simulink model "GS_model"  (R2018b)
settings: Solver=ode5  StartTime=0.0  StopTime=SimuStopTime  FixedStep=T_Simu  RelTol=1e-3
InitFcn:
  | Initial
undefined symbols (not defined in the file or in its folder): Aba10, Aba20, aeroCIP2006_S, aeroCIP2006_X, aeroCIP2006_Y, Agl0, Ass_kS, Ass_n1, Ass_n2, Ass_n3, Ass_n4, Ass_Noise, Ass_R, Ass_Resolution, Ass_TmOrder, AssA_Fix_Abs, AssB_Fix_Abs, AssC_Fix_Abs, AssD_Fix_Abs, AssE_Fix_Aps, AssF_Fix_Aps, C, c_max, c_min, Cd, CenterOfFigNX, CenterOfFigNY, CenterOfFigNZ, CenterOfFigP1, CenterOfFigP2, CenterOfFigPX, CenterOfFigPY, CenterOfFigPZ, Cmu, Crou, DEG2RAD, DiscIntNeverNeededParam, Eg_Dir, Eg_F, Eg_PrepareTime, Eg_r_L_L, Fw_Abf, Fw_Hmax, Fw_J, Fw_Spd0, Fw_Tmax, git_hash_BaseLine, git_hash_Project, Gnss_Noise_Pos, Gnss_Noise_Vel, Gnss_PropgationTime, GyroA_Fix_Abg, GyroA_Noise, GyroB_Fix_Abg, GyroB_Noise, GyroC_Fix_Abg, GyroC_Noise, GyroD_Fix_Abg, GyroD_Noise, h ... (+94)
libraries: simulink x308, sharedutil x46, aerolibutil x37, sharedtransform x31, vrlib x14, aerolibgravity2 x2
(part 10 of 20)

== system GS_model/Subsystem2/Subsystem/Actuator/FlyWheel/FwAModel4/FWMath&ErrModel/Subsystem1 ==
  Fb_FW_T : Inport
  TC_FW_TSet : Inport  Port=2
  FWNum : Inport  Port=3
  TC_FWErr_TOp : Inport  Port=4
  Compare To Constant : simulink/Logic and Bit Operations/Compare To Constant  relop===  const=0  OutDataTypeStr=boolean
  Compare To Constant1 : simulink/Logic and Bit Operations/Compare To Constant  relop===  const=0  OutDataTypeStr=boolean
  Demux : Demux  Outputs=[1;2]
  Demux1 : Demux  Outputs=2
  Demux2 : Demux  Outputs=2
  If : If  IfExpression=u1 == 1
  If Action Subsystem : Subsystem  TreatAsAtomicUnit=on
  If Action Subsystem1 : Subsystem  TreatAsAtomicUnit=on
  Logical Operator : Logic  Operator=OR  AllPortsSameDT=off  OutDataTypeStr=boolean
  Logical Operator1 : Logic  Operator=OR  AllPortsSameDT=off  OutDataTypeStr=boolean
  Merge : Merge
  Relational Operator1 : RelationalOperator  Operator===  OutDataTypeStr=boolean  RndMeth=Simplest
  Relational Operator3 : RelationalOperator  Operator===  OutDataTypeStr=boolean  RndMeth=Simplest
  Sum : Sum  Inputs=|++
  Triggered Subsystem1 : Subsystem  TreatAsAtomicUnit=on
      mask Display: disp('FWChoice')
  Triggered Subsystem2 : Subsystem  TreatAsAtomicUnit=on
      mask Display: disp('FWChoice')
  TM_FW_T : Outport
  wires:
  FWNum/1 -> Relational Operator3/1, Relational Operator1/1
  Compare To Constant1/1 -> Logical Operator1/1
  Relational Operator1/1 -> Logical Operator1/2
  Demux2/1 -> Compare To Constant1/1, Relational Operator1/2
  Logical Operator1/1 -> Triggered Subsystem2/Enable
  Logical Operator/1 -> Triggered Subsystem1/Enable
  Demux/1 -> Relational Operator3/2, Compare To Constant/1
  Relational Operator3/1 -> Logical Operator/2
  Compare To Constant/1 -> Logical Operator/1
  Demux1/1 -> If/1
  If Action Subsystem/1(Out1) -> Merge/1
  Triggered Subsystem1/1(Out1) -> Demux1/1
  Demux/2 -> Triggered Subsystem1/1(In1)
  If/1 -> If Action Subsystem/Action
  TC_FW_TSet/1 -> Demux/1
  Sum/1 -> If Action Subsystem1/1(In1)
  Merge/1 -> TM_FW_T/1
  TC_FWErr_TOp/1 -> Demux2/1
  Demux2/2 -> Triggered Subsystem2/1(In1)
  Triggered Subsystem2/1(Out1) -> Sum/1
  If Action Subsystem1/1(Out1) -> Merge/2
  Demux1/2 -> If Action Subsystem/1(In1)
  If/2 -> If Action Subsystem1/Action
  Fb_FW_T/1 -> Sum/2

== system GS_model/Subsystem2/Subsystem/Actuator/FlyWheel/FwAModel4/FWMath&ErrModel/Subsystem2 ==
  Fb_FW_Spd : Inport
  TC_FW_SpdSet : Inport  Port=2
  FWNum : Inport  Port=3
  TC_FWErr_SpdOp : Inport  Port=4
  Compare To Constant : simulink/Logic and Bit Operations/Compare To Constant  relop===  const=0  OutDataTypeStr=boolean
  Compare To Constant1 : simulink/Logic and Bit Operations/Compare To Constant  relop===  const=0  OutDataTypeStr=boolean
  Demux : Demux  Outputs=[1;2]
  Demux1 : Demux  Outputs=2
  Demux2 : Demux  Outputs=2
  If : If  IfExpression=u1 == 1
  If Action Subsystem : Subsystem  TreatAsAtomicUnit=on
  If Action Subsystem1 : Subsystem  TreatAsAtomicUnit=on
  Logical Operator : Logic  Operator=OR  AllPortsSameDT=off  OutDataTypeStr=boolean
  Logical Operator1 : Logic  Operator=OR  AllPortsSameDT=off  OutDataTypeStr=boolean
  Merge : Merge
  Relational Operator1 : RelationalOperator  Operator===  OutDataTypeStr=boolean  RndMeth=Simplest
  Relational Operator2 : RelationalOperator  Operator===  OutDataTypeStr=boolean  RndMeth=Simplest
  Sum : Sum  Inputs=|++
  Triggered Subsystem1 : Subsystem  TreatAsAtomicUnit=on
      mask Display: disp('FWChoice')
  Triggered Subsystem2 : Subsystem  TreatAsAtomicUnit=on
      mask Display: disp('FWChoice')
  TM_FW_Spd : Outport
  wires:
  Logical Operator1/1 -> Triggered Subsystem2/Enable
  Compare To Constant1/1 -> Logical Operator1/1
  Relational Operator2/1 -> Logical Operator1/2
  Logical Operator/1 -> Triggered Subsystem1/Enable
  Compare To Constant/1 -> Logical Operator/1
  Relational Operator1/1 -> Logical Operator/2
  If/2 -> If Action Subsystem1/Action
  If Action Subsystem/1(Out1) -> Merge/1
  Demux2/1 -> Relational Operator2/2, Compare To Constant1/1
  FWNum/1 -> Relational Operator1/1, Relational Operator2/1
  Triggered Subsystem1/1(Out1) -> Demux1/1
  Fb_FW_Spd/1 -> Sum/2
  Demux/2 -> Triggered Subsystem1/1(In1)
  If Action Subsystem1/1(Out1) -> Merge/2
  Demux1/1 -> If/1
  Demux2/2 -> Triggered Subsystem2/1(In1)
  Demux1/2 -> If Action Subsystem/1(In1)
  Sum/1 -> If Action Subsystem1/1(In1)
  Triggered Subsystem2/1(Out1) -> Sum/1
  TC_FWErr_SpdOp/1 -> Demux2/1
  If/1 -> If Action Subsystem/Action
  Merge/1 -> TM_FW_Spd/1
  Demux/1 -> Relational Operator1/2, Compare To Constant/1
  TC_FW_SpdSet/1 -> Demux/1

== system GS_model/Subsystem2/Subsystem/Actuator/FlyWheel/FwAModel4/FWMath&ErrModel/Subsystem4 ==
  FWNum : Inport
  FW_Mode : Inport  Port=2
  TC_FW_ModeSet : Inport  Port=3
  Compare To Constant : simulink/Logic and Bit Operations/Compare To Constant  relop===  const=0  OutDataTypeStr=boolean
  Demux : Demux  Outputs=[1;2]
  Demux1 : Demux  Outputs=2
  If : If  IfExpression=u1 == 1
  If Action Subsystem : Subsystem  TreatAsAtomicUnit=on
  If Action Subsystem1 : Subsystem  TreatAsAtomicUnit=on
  Logical Operator : Logic  Operator=OR  AllPortsSameDT=off  OutDataTypeStr=boolean
  Merge : Merge
  Relational Operator1 : RelationalOperator  Operator===  OutDataTypeStr=boolean  RndMeth=Simplest
  Triggered Subsystem1 : Subsystem  TreatAsAtomicUnit=on
      mask Display: disp('FWChoice')
  Fb_FW_Mode : Outport
  wires:
  Compare To Constant/1 -> Logical Operator/1
  Logical Operator/1 -> Triggered Subsystem1/Enable
  Relational Operator1/1 -> Logical Operator/2
  TC_FW_ModeSet/1 -> Demux/1
  FWNum/1 -> Relational Operator1/1
  Demux/2 -> Triggered Subsystem1/1(In1)
  Demux/1 -> Relational Operator1/2, Compare To Constant/1
  Demux1/1 -> If/1
  If/1 -> If Action Subsystem/Action
  Demux1/2 -> If Action Subsystem/1(In1)
  Triggered Subsystem1/1(Out1) -> Demux1/1
  If/2 -> If Action Subsystem1/Action
  FW_Mode/1 -> If Action Subsystem1/1(In1)
  If Action Subsystem/1(Out1) -> Merge/1
  If Action Subsystem1/1(Out1) -> Merge/2
  Merge/1 -> Fb_FW_Mode/1

== system GS_model/Subsystem2/Subsystem/Actuator/FlyWheel/FwAModel5/FWDataSourceChoice/DelayModel ==
  TC_FW_Delay : Inport
  FW_Cmd_Mode : Inport  Port=2
  FW_Cmd_Spd : Inport  Port=3
  FW_Cmd_T : Inport  Port=4
  Constant3 : Constant
  Sum8 : Sum  Inputs=|++
  delay1 : Subsystem
  delay2 : Subsystem
  delay3 : Subsystem
  Cmd_Mode : Outport
  Cmd_Spd : Outport  Port=2
  Cmd_T : Outport  Port=3
  wires:
  delay2/1(Out1) -> Cmd_T/1
  FW_Cmd_T/1 -> delay2/2(In2)
  delay1/1(Out1) -> Cmd_Spd/1
  Sum8/1 -> delay1/1(In1), delay2/1(In1), delay3/1(In1)
  FW_Cmd_Spd/1 -> delay1/2(In2)
  Constant3/1 -> Sum8/2
  TC_FW_Delay/1 -> Sum8/1
  FW_Cmd_Mode/1 -> delay3/2(In2)
  delay3/1(Out1) -> Cmd_Mode/1

== system GS_model/Subsystem2/Subsystem/Actuator/FlyWheel/FwAModel5/FWMath&ErrModel/Subsystem1 ==
  Fb_FW_T : Inport
  TC_FW_TSet : Inport  Port=2
  FWNum : Inport  Port=3
  TC_FWErr_TOp : Inport  Port=4
  Compare To Constant : simulink/Logic and Bit Operations/Compare To Constant  relop===  const=0  OutDataTypeStr=boolean
  Compare To Constant1 : simulink/Logic and Bit Operations/Compare To Constant  relop===  const=0  OutDataTypeStr=boolean
  Demux : Demux  Outputs=[1;2]
  Demux1 : Demux  Outputs=2
  Demux2 : Demux  Outputs=2
  If : If  IfExpression=u1 == 1
  If Action Subsystem : Subsystem  TreatAsAtomicUnit=on
  If Action Subsystem1 : Subsystem  TreatAsAtomicUnit=on
  Logical Operator : Logic  Operator=OR  AllPortsSameDT=off  OutDataTypeStr=boolean
  Logical Operator1 : Logic  Operator=OR  AllPortsSameDT=off  OutDataTypeStr=boolean
  Merge : Merge
  Relational Operator1 : RelationalOperator  Operator===  OutDataTypeStr=boolean  RndMeth=Simplest
  Relational Operator3 : RelationalOperator  Operator===  OutDataTypeStr=boolean  RndMeth=Simplest
  Sum : Sum  Inputs=|++
  Triggered Subsystem1 : Subsystem  TreatAsAtomicUnit=on
      mask Display: disp('FWChoice')
  Triggered Subsystem2 : Subsystem  TreatAsAtomicUnit=on
      mask Display: disp('FWChoice')
  TM_FW_T : Outport
  wires:
  Fb_FW_T/1 -> Sum/2
  If/2 -> If Action Subsystem1/Action
  Demux1/2 -> If Action Subsystem/1(In1)
  If Action Subsystem1/1(Out1) -> Merge/2
  Triggered Subsystem2/1(Out1) -> Sum/1
  Demux2/2 -> Triggered Subsystem2/1(In1)
  TC_FWErr_TOp/1 -> Demux2/1
  Merge/1 -> TM_FW_T/1
  Sum/1 -> If Action Subsystem1/1(In1)
  TC_FW_TSet/1 -> Demux/1
  If/1 -> If Action Subsystem/Action
  Demux/2 -> Triggered Subsystem1/1(In1)
  Triggered Subsystem1/1(Out1) -> Demux1/1
  If Action Subsystem/1(Out1) -> Merge/1
  Demux1/1 -> If/1
  Compare To Constant/1 -> Logical Operator/1
  Relational Operator3/1 -> Logical Operator/2
  Demux/1 -> Compare To Constant/1, Relational Operator3/2
  Logical Operator/1 -> Triggered Subsystem1/Enable
  Logical Operator1/1 -> Triggered Subsystem2/Enable
  Demux2/1 -> Relational Operator1/2, Compare To Constant1/1
  Relational Operator1/1 -> Logical Operator1/2
  Compare To Constant1/1 -> Logical Operator1/1
  FWNum/1 -> Relational Operator1/1, Relational Operator3/1

== system GS_model/Subsystem2/Subsystem/Actuator/FlyWheel/FwAModel5/FWMath&ErrModel/Subsystem2 ==
  Fb_FW_Spd : Inport
  TC_FW_SpdSet : Inport  Port=2
  FWNum : Inport  Port=3
  TC_FWErr_SpdOp : Inport  Port=4
  Compare To Constant : simulink/Logic and Bit Operations/Compare To Constant  relop===  const=0  OutDataTypeStr=boolean
  Compare To Constant1 : simulink/Logic and Bit Operations/Compare To Constant  relop===  const=0  OutDataTypeStr=boolean
  Demux : Demux  Outputs=[1;2]
  Demux1 : Demux  Outputs=2
  Demux2 : Demux  Outputs=2
  If : If  IfExpression=u1 == 1
  If Action Subsystem : Subsystem  TreatAsAtomicUnit=on
  If Action Subsystem1 : Subsystem  TreatAsAtomicUnit=on
  Logical Operator : Logic  Operator=OR  AllPortsSameDT=off  OutDataTypeStr=boolean
  Logical Operator1 : Logic  Operator=OR  AllPortsSameDT=off  OutDataTypeStr=boolean
  Merge : Merge
  Relational Operator1 : RelationalOperator  Operator===  OutDataTypeStr=boolean  RndMeth=Simplest
  Relational Operator2 : RelationalOperator  Operator===  OutDataTypeStr=boolean  RndMeth=Simplest
  Sum : Sum  Inputs=|++
  Triggered Subsystem1 : Subsystem  TreatAsAtomicUnit=on
      mask Display: disp('FWChoice')
  Triggered Subsystem2 : Subsystem  TreatAsAtomicUnit=on
      mask Display: disp('FWChoice')
  TM_FW_Spd : Outport
  wires:
  TC_FW_SpdSet/1 -> Demux/1
  Demux/1 -> Compare To Constant/1, Relational Operator1/2
  Merge/1 -> TM_FW_Spd/1
  If/1 -> If Action Subsystem/Action
  TC_FWErr_SpdOp/1 -> Demux2/1
  Triggered Subsystem2/1(Out1) -> Sum/1
  Sum/1 -> If Action Subsystem1/1(In1)
  Demux1/2 -> If Action Subsystem/1(In1)
  Demux2/2 -> Triggered Subsystem2/1(In1)
  Demux1/1 -> If/1
  If Action Subsystem1/1(Out1) -> Merge/2
  Demux/2 -> Triggered Subsystem1/1(In1)
  Fb_FW_Spd/1 -> Sum/2
  Triggered Subsystem1/1(Out1) -> Demux1/1
  FWNum/1 -> Relational Operator2/1, Relational Operator1/1
  Demux2/1 -> Compare To Constant1/1, Relational Operator2/2
  If Action Subsystem/1(Out1) -> Merge/1
  If/2 -> If Action Subsystem1/Action
  Relational Operator1/1 -> Logical Operator/2
  Compare To Constant/1 -> Logical Operator/1
  Logical Operator/1 -> Triggered Subsystem1/Enable
  Relational Operator2/1 -> Logical Operator1/2
  Compare To Constant1/1 -> Logical Operator1/1
  Logical Operator1/1 -> Triggered Subsystem2/Enable

== system GS_model/Subsystem2/Subsystem/Actuator/FlyWheel/FwAModel5/FWMath&ErrModel/Subsystem4 ==
  FWNum : Inport
  FW_Mode : Inport  Port=2
  TC_FW_ModeSet : Inport  Port=3
  Compare To Constant : simulink/Logic and Bit Operations/Compare To Constant  relop===  const=0  OutDataTypeStr=boolean
  Demux : Demux  Outputs=[1;2]
  Demux1 : Demux  Outputs=2
  If : If  IfExpression=u1 == 1
  If Action Subsystem : Subsystem  TreatAsAtomicUnit=on
  If Action Subsystem1 : Subsystem  TreatAsAtomicUnit=on
  Logical Operator : Logic  Operator=OR  AllPortsSameDT=off  OutDataTypeStr=boolean
  Merge : Merge
  Relational Operator1 : RelationalOperator  Operator===  OutDataTypeStr=boolean  RndMeth=Simplest
  Triggered Subsystem1 : Subsystem  TreatAsAtomicUnit=on
      mask Display: disp('FWChoice')
  Fb_FW_Mode : Outport
  wires:
  Merge/1 -> Fb_FW_Mode/1
  If Action Subsystem1/1(Out1) -> Merge/2
  If Action Subsystem/1(Out1) -> Merge/1
  FW_Mode/1 -> If Action Subsystem1/1(In1)
  If/2 -> If Action Subsystem1/Action
  Triggered Subsystem1/1(Out1) -> Demux1/1
  Demux1/2 -> If Action Subsystem/1(In1)
  If/1 -> If Action Subsystem/Action
  Demux1/1 -> If/1
  Demux/1 -> Compare To Constant/1, Relational Operator1/2
  Demux/2 -> Triggered Subsystem1/1(In1)
  FWNum/1 -> Relational Operator1/1
  TC_FW_ModeSet/1 -> Demux/1
  Relational Operator1/1 -> Logical Operator/2
  Logical Operator/1 -> Triggered Subsystem1/Enable
  Compare To Constant/1 -> Logical Operator/1

== system GS_model/Subsystem2/Subsystem/Actuator/FlyWheel/FwAModel6/FWDataSourceChoice/DelayModel ==
  TC_FW_Delay : Inport
  FW_Cmd_Mode : Inport  Port=2
  FW_Cmd_Spd : Inport  Port=3
  FW_Cmd_T : Inport  Port=4
  Constant3 : Constant
  Sum8 : Sum  Inputs=|++
  delay1 : Subsystem
  delay2 : Subsystem
  delay3 : Subsystem
  Cmd_Mode : Outport
  Cmd_Spd : Outport  Port=2
  Cmd_T : Outport  Port=3
  wires:
  delay3/1(Out1) -> Cmd_Mode/1
  FW_Cmd_Mode/1 -> delay3/2(In2)
  TC_FW_Delay/1 -> Sum8/1
  Constant3/1 -> Sum8/2
  FW_Cmd_Spd/1 -> delay1/2(In2)
  Sum8/1 -> delay3/1(In1), delay2/1(In1), delay1/1(In1)
  delay1/1(Out1) -> Cmd_Spd/1
  FW_Cmd_T/1 -> delay2/2(In2)
  delay2/1(Out1) -> Cmd_T/1

== system GS_model/Subsystem2/Subsystem/Actuator/FlyWheel/FwAModel6/FWMath&ErrModel/Subsystem1 ==
  Fb_FW_T : Inport
  TC_FW_TSet : Inport  Port=2
  FWNum : Inport  Port=3
  TC_FWErr_TOp : Inport  Port=4
  Compare To Constant : simulink/Logic and Bit Operations/Compare To Constant  relop===  const=0  OutDataTypeStr=boolean
  Compare To Constant1 : simulink/Logic and Bit Operations/Compare To Constant  relop===  const=0  OutDataTypeStr=boolean
  Demux : Demux  Outputs=[1;2]
  Demux1 : Demux  Outputs=2
  Demux2 : Demux  Outputs=2
  If : If  IfExpression=u1 == 1
  If Action Subsystem : Subsystem  TreatAsAtomicUnit=on
  If Action Subsystem1 : Subsystem  TreatAsAtomicUnit=on
  Logical Operator : Logic  Operator=OR  AllPortsSameDT=off  OutDataTypeStr=boolean
  Logical Operator1 : Logic  Operator=OR  AllPortsSameDT=off  OutDataTypeStr=boolean
  Merge : Merge
  Relational Operator1 : RelationalOperator  Operator===  OutDataTypeStr=boolean  RndMeth=Simplest
  Relational Operator3 : RelationalOperator  Operator===  OutDataTypeStr=boolean  RndMeth=Simplest
  Sum : Sum  Inputs=|++
  Triggered Subsystem1 : Subsystem  TreatAsAtomicUnit=on
      mask Display: disp('FWChoice')
  Triggered Subsystem2 : Subsystem  TreatAsAtomicUnit=on
      mask Display: disp('FWChoice')
  TM_FW_T : Outport
  wires:
  FWNum/1 -> Relational Operator3/1, Relational Operator1/1
  Compare To Constant1/1 -> Logical Operator1/1
  Relational Operator1/1 -> Logical Operator1/2
  Demux2/1 -> Compare To Constant1/1, Relational Operator1/2
  Logical Operator1/1 -> Triggered Subsystem2/Enable
  Logical Operator/1 -> Triggered Subsystem1/Enable
  Demux/1 -> Relational Operator3/2, Compare To Constant/1
  Relational Operator3/1 -> Logical Operator/2
  Compare To Constant/1 -> Logical Operator/1
  Demux1/1 -> If/1
  If Action Subsystem/1(Out1) -> Merge/1
  Triggered Subsystem1/1(Out1) -> Demux1/1
  Demux/2 -> Triggered Subsystem1/1(In1)
  If/1 -> If Action Subsystem/Action
  TC_FW_TSet/1 -> Demux/1
  Sum/1 -> If Action Subsystem1/1(In1)
  Merge/1 -> TM_FW_T/1
  TC_FWErr_TOp/1 -> Demux2/1
  Demux2/2 -> Triggered Subsystem2/1(In1)
  Triggered Subsystem2/1(Out1) -> Sum/1
  If Action Subsystem1/1(Out1) -> Merge/2
  Demux1/2 -> If Action Subsystem/1(In1)
  If/2 -> If Action Subsystem1/Action
  Fb_FW_T/1 -> Sum/2

== system GS_model/Subsystem2/Subsystem/Actuator/FlyWheel/FwAModel6/FWMath&ErrModel/Subsystem2 ==
  Fb_FW_Spd : Inport
  TC_FW_SpdSet : Inport  Port=2
  FWNum : Inport  Port=3
  TC_FWErr_SpdOp : Inport  Port=4
  Compare To Constant : simulink/Logic and Bit Operations/Compare To Constant  relop===  const=0  OutDataTypeStr=boolean
  Compare To Constant1 : simulink/Logic and Bit Operations/Compare To Constant  relop===  const=0  OutDataTypeStr=boolean
  Demux : Demux  Outputs=[1;2]
  Demux1 : Demux  Outputs=2
  Demux2 : Demux  Outputs=2
  If : If  IfExpression=u1 == 1
  If Action Subsystem : Subsystem  TreatAsAtomicUnit=on
  If Action Subsystem1 : Subsystem  TreatAsAtomicUnit=on
  Logical Operator : Logic  Operator=OR  AllPortsSameDT=off  OutDataTypeStr=boolean
  Logical Operator1 : Logic  Operator=OR  AllPortsSameDT=off  OutDataTypeStr=boolean
  Merge : Merge
  Relational Operator1 : RelationalOperator  Operator===  OutDataTypeStr=boolean  RndMeth=Simplest
  Relational Operator2 : RelationalOperator  Operator===  OutDataTypeStr=boolean  RndMeth=Simplest
  Sum : Sum  Inputs=|++
  Triggered Subsystem1 : Subsystem  TreatAsAtomicUnit=on
      mask Display: disp('FWChoice')
  Triggered Subsystem2 : Subsystem  TreatAsAtomicUnit=on
      mask Display: disp('FWChoice')
  TM_FW_Spd : Outport
  wires:
  Logical Operator1/1 -> Triggered Subsystem2/Enable
  Compare To Constant1/1 -> Logical Operator1/1
  Relational Operator2/1 -> Logical Operator1/2
  Logical Operator/1 -> Triggered Subsystem1/Enable
  Compare To Constant/1 -> Logical Operator/1
  Relational Operator1/1 -> Logical Operator/2
  If/2 -> If Action Subsystem1/Action
  If Action Subsystem/1(Out1) -> Merge/1
  Demux2/1 -> Relational Operator2/2, Compare To Constant1/1
  FWNum/1 -> Relational Operator1/1, Relational Operator2/1
  Triggered Subsystem1/1(Out1) -> Demux1/1
  Fb_FW_Spd/1 -> Sum/2
  Demux/2 -> Triggered Subsystem1/1(In1)
  If Action Subsystem1/1(Out1) -> Merge/2
  Demux1/1 -> If/1
  Demux2/2 -> Triggered Subsystem2/1(In1)
  Demux1/2 -> If Action Subsystem/1(In1)
  Sum/1 -> If Action Subsystem1/1(In1)
  Triggered Subsystem2/1(Out1) -> Sum/1
  TC_FWErr_SpdOp/1 -> Demux2/1
  If/1 -> If Action Subsystem/Action
  Merge/1 -> TM_FW_Spd/1
  Demux/1 -> Relational Operator1/2, Compare To Constant/1
  TC_FW_SpdSet/1 -> Demux/1

== system GS_model/Subsystem2/Subsystem/Actuator/FlyWheel/FwAModel6/FWMath&ErrModel/Subsystem4 ==
  FWNum : Inport
  FW_Mode : Inport  Port=2
  TC_FW_ModeSet : Inport  Port=3
  Compare To Constant : simulink/Logic and Bit Operations/Compare To Constant  relop===  const=0  OutDataTypeStr=boolean
  Demux : Demux  Outputs=[1;2]
  Demux1 : Demux  Outputs=2
  If : If  IfExpression=u1 == 1
  If Action Subsystem : Subsystem  TreatAsAtomicUnit=on
  If Action Subsystem1 : Subsystem  TreatAsAtomicUnit=on
  Logical Operator : Logic  Operator=OR  AllPortsSameDT=off  OutDataTypeStr=boolean
  Merge : Merge
  Relational Operator1 : RelationalOperator  Operator===  OutDataTypeStr=boolean  RndMeth=Simplest
  Triggered Subsystem1 : Subsystem  TreatAsAtomicUnit=on
      mask Display: disp('FWChoice')
  Fb_FW_Mode : Outport
  wires:
  Compare To Constant/1 -> Logical Operator/1
  Logical Operator/1 -> Triggered Subsystem1/Enable
  Relational Operator1/1 -> Logical Operator/2
  TC_FW_ModeSet/1 -> Demux/1
  FWNum/1 -> Relational Operator1/1
  Demux/2 -> Triggered Subsystem1/1(In1)
  Demux/1 -> Relational Operator1/2, Compare To Constant/1
  Demux1/1 -> If/1
  If/1 -> If Action Subsystem/Action
  Demux1/2 -> If Action Subsystem/1(In1)
  Triggered Subsystem1/1(Out1) -> Demux1/1
  If/2 -> If Action Subsystem1/Action
  FW_Mode/1 -> If Action Subsystem1/1(In1)
  If Action Subsystem/1(Out1) -> Merge/1
  If Action Subsystem1/1(Out1) -> Merge/2
  Merge/1 -> Fb_FW_Mode/1

== system GS_model/Subsystem2/Subsystem/Actuator/Magnetorquer/Mt_MathModel/MtA1/>=<0 to 012 ==
  note: 1--正向
  note: 0
  note: 2--负向
  In1 : Inport
  Add1 : Sum  Inputs=+++
  Cast To Double : DataTypeConversion  OutDataTypeStr=double
  Cast To Double1 : DataTypeConversion  OutDataTypeStr=double
  Cast To Double2 : DataTypeConversion  OutDataTypeStr=double
  Compare To Zero : simulink/Logic and Bit Operations/Compare To Zero  relop=<  OutDataTypeStr=boolean
  Compare To Zero1 : simulink/Logic and Bit Operations/Compare To Zero  relop===  OutDataTypeStr=boolean
  Compare To Zero2 : simulink/Logic and Bit Operations/Compare To Zero  relop=>  OutDataTypeStr=boolean
  Constant1 : Constant
  Constant2 : Constant  Value=0
  Constant20 : Constant  Value=2
  Product1 : Product  SaturateOnIntegerOverflow=on  OutDataTypeStr=Inherit: Same as first input
  Product2 : Product  SaturateOnIntegerOverflow=on  OutDataTypeStr=Inherit: Same as first input
  Product6 : Product  SaturateOnIntegerOverflow=on  OutDataTypeStr=Inherit: Same as first input
  Out1 : Outport
  wires:
  Product1/1 -> Add1/2
  Product6/1 -> Add1/1
  Compare To Zero1/1 -> Cast To Double1/1
  Constant2/1 -> Product1/1
  In1/1 -> Compare To Zero2/1, Compare To Zero1/1, Compare To Zero/1
  Compare To Zero/1 -> Cast To Double/1
  Compare To Zero2/1 -> Cast To Double2/1
  Add1/1 -> Out1/1
  Cast To Double/1 -> Product6/2
  Cast To Double1/1 -> Product1/2
  Constant20/1 -> Product6/1
  Constant1/1 -> Product2/1
  Cast To Double2/1 -> Product2/2
  Product2/1 -> Add1/3

== system GS_model/Subsystem2/Subsystem/Actuator/Magnetorquer/Mt_MathModel/MtA1/If Action Subsystem3 ==
  In1 : Inport
  Action Port : ActionPort  ActionType=else
  Out1 : Outport
  wires:
  In1/1 -> Out1/1

== system GS_model/Subsystem2/Subsystem/Actuator/Magnetorquer/Mt_MathModel/MtA1/If Action Subsystem4 ==
  In1 : Inport
  Action Port : ActionPort  ActionType=then
  Out1 : Outport
  wires:
  In1/1 -> Out1/1

== system GS_model/Subsystem2/Subsystem/Actuator/Magnetorquer/Mt_MathModel/MtA1/Mag_CmdCal ==
  Cmd_Dir : Inport
  Cmd_Cur : Inport  Port=2
  55/AA to +/- : Subsystem
  >=<0 to 012 : Subsystem
  Product1 : Product
  Transfer Fcn : TransferFcn  Denominator=[Tao_Mt/3 1]
  "Cmd_Curr " : Outport
  Cmd_Dirr : Outport  Port=2
  wires:
  Cmd_Cur/1 -> Product1/1
  55/AA to +/-/1(Out1) -> >=<0 to 012/1(In1), Product1/2
  Product1/1 -> Transfer Fcn/1  "Mag_current"
  Cmd_Dir/1 -> 55/AA to +/-/1(In1)
  >=<0 to 012/1(Out1) -> Cmd_Dirr/1
  Transfer Fcn/1 -> "Cmd_Curr "/1

== system GS_model/Subsystem2/Subsystem/Actuator/Magnetorquer/Mt_MathModel/MtA1/Triggered Subsystem6 ==
  In1 : Inport
  Enable : EnablePort
  Out1 : Outport  InitialOutput=0
  wires:
  In1/1 -> Out1/1

== system GS_model/Subsystem2/Subsystem/Actuator/Magnetorquer/Mt_MathModel/MtA2/>=<0 to 012 ==
  note: 2--负向
  note: 0
  note: 1--正向
  In1 : Inport
  Add1 : Sum  Inputs=+++
  Cast To Double : DataTypeConversion  OutDataTypeStr=double
  Cast To Double1 : DataTypeConversion  OutDataTypeStr=double
  Cast To Double2 : DataTypeConversion  OutDataTypeStr=double
  Compare To Zero : simulink/Logic and Bit Operations/Compare To Zero  relop=<  OutDataTypeStr=boolean
  Compare To Zero1 : simulink/Logic and Bit Operations/Compare To Zero  relop===  OutDataTypeStr=boolean
  Compare To Zero2 : simulink/Logic and Bit Operations/Compare To Zero  relop=>  OutDataTypeStr=boolean
  Constant1 : Constant
  Constant2 : Constant  Value=0
  Constant20 : Constant  Value=2
  Product1 : Product  SaturateOnIntegerOverflow=on  OutDataTypeStr=Inherit: Same as first input
  Product2 : Product  SaturateOnIntegerOverflow=on  OutDataTypeStr=Inherit: Same as first input
  Product6 : Product  SaturateOnIntegerOverflow=on  OutDataTypeStr=Inherit: Same as first input
  Out1 : Outport
  wires:
  Product2/1 -> Add1/3
  Cast To Double2/1 -> Product2/2
  Constant1/1 -> Product2/1
  Constant20/1 -> Product6/1
  Cast To Double1/1 -> Product1/2
  Cast To Double/1 -> Product6/2
  Add1/1 -> Out1/1
  Compare To Zero2/1 -> Cast To Double2/1
  Compare To Zero/1 -> Cast To Double/1
  In1/1 -> Compare To Zero/1, Compare To Zero1/1, Compare To Zero2/1
  Constant2/1 -> Product1/1
  Compare To Zero1/1 -> Cast To Double1/1
  Product6/1 -> Add1/1
  Product1/1 -> Add1/2

== system GS_model/Subsystem2/Subsystem/Actuator/Magnetorquer/Mt_MathModel/MtA2/If Action Subsystem3 ==
  In1 : Inport
  Action Port : ActionPort  ActionType=else
  Out1 : Outport
  wires:
  In1/1 -> Out1/1

== system GS_model/Subsystem2/Subsystem/Actuator/Magnetorquer/Mt_MathModel/MtA2/If Action Subsystem4 ==
  In1 : Inport
  Action Port : ActionPort  ActionType=then
  Out1 : Outport
  wires:
  In1/1 -> Out1/1

== system GS_model/Subsystem2/Subsystem/Actuator/Magnetorquer/Mt_MathModel/MtA2/Mag_CmdCal ==
  Cmd_Dir : Inport
  Cmd_Cur : Inport  Port=2
  55/AA to +/- : Subsystem
  >=<0 to 012 : Subsystem
  Product1 : Product
  Transfer Fcn : TransferFcn  Denominator=[Tao_Mt/3 1]
  "Cmd_Curr " : Outport
  Cmd_Dirr : Outport  Port=2
  wires:
  Transfer Fcn/1 -> "Cmd_Curr "/1
  >=<0 to 012/1(Out1) -> Cmd_Dirr/1
  Cmd_Dir/1 -> 55/AA to +/-/1(In1)
  Product1/1 -> Transfer Fcn/1  "Mag_current"
  55/AA to +/-/1(Out1) -> Product1/2, >=<0 to 012/1(In1)
  Cmd_Cur/1 -> Product1/1

== system GS_model/Subsystem2/Subsystem/Actuator/Magnetorquer/Mt_MathModel/MtA2/Triggered Subsystem6 ==
  In1 : Inport
  Enable : EnablePort
  Out1 : Outport  InitialOutput=0
  wires:
  In1/1 -> Out1/1

== system GS_model/Subsystem2/Subsystem/Actuator/Magnetorquer/Mt_MathModel/MtA3/>=<0 to 012 ==
  note: 1--正向
  note: 0
  note: 2--负向
  In1 : Inport
  Add1 : Sum  Inputs=+++
  Cast To Double : DataTypeConversion  OutDataTypeStr=double
  Cast To Double1 : DataTypeConversion  OutDataTypeStr=double
  Cast To Double2 : DataTypeConversion  OutDataTypeStr=double
  Compare To Zero : simulink/Logic and Bit Operations/Compare To Zero  relop=<  OutDataTypeStr=boolean
  Compare To Zero1 : simulink/Logic and Bit Operations/Compare To Zero  relop===  OutDataTypeStr=boolean
  Compare To Zero2 : simulink/Logic and Bit Operations/Compare To Zero  relop=>  OutDataTypeStr=boolean
  Constant1 : Constant
  Constant2 : Constant  Value=0
  Constant20 : Constant  Value=2
  Product1 : Product  SaturateOnIntegerOverflow=on  OutDataTypeStr=Inherit: Same as first input
  Product2 : Product  SaturateOnIntegerOverflow=on  OutDataTypeStr=Inherit: Same as first input
  Product6 : Product  SaturateOnIntegerOverflow=on  OutDataTypeStr=Inherit: Same as first input
  Out1 : Outport
  wires:
  Product1/1 -> Add1/2
  Product6/1 -> Add1/1
  Compare To Zero1/1 -> Cast To Double1/1
  Constant2/1 -> Product1/1
  In1/1 -> Compare To Zero2/1, Compare To Zero1/1, Compare To Zero/1
  Compare To Zero/1 -> Cast To Double/1
  Compare To Zero2/1 -> Cast To Double2/1
  Add1/1 -> Out1/1
  Cast To Double/1 -> Product6/2
  Cast To Double1/1 -> Product1/2
  Constant20/1 -> Product6/1
  Constant1/1 -> Product2/1
  Cast To Double2/1 -> Product2/2
  Product2/1 -> Add1/3

== system GS_model/Subsystem2/Subsystem/Actuator/Magnetorquer/Mt_MathModel/MtA3/If Action Subsystem3 ==
  In1 : Inport
  Action Port : ActionPort  ActionType=else
  Out1 : Outport
  wires:
  In1/1 -> Out1/1

== system GS_model/Subsystem2/Subsystem/Actuator/Magnetorquer/Mt_MathModel/MtA3/If Action Subsystem4 ==
  In1 : Inport
  Action Port : ActionPort  ActionType=then
  Out1 : Outport
  wires:
  In1/1 -> Out1/1

== system GS_model/Subsystem2/Subsystem/Actuator/Magnetorquer/Mt_MathModel/MtA3/Mag_CmdCal ==
  Cmd_Dir : Inport
  Cmd_Cur : Inport  Port=2
  55/AA to +/- : Subsystem
  >=<0 to 012 : Subsystem
  Product1 : Product
  Transfer Fcn : TransferFcn  Denominator=[Tao_Mt/3 1]
  "Cmd_Curr " : Outport
  Cmd_Dirr : Outport  Port=2
  wires:
  Cmd_Cur/1 -> Product1/1
  55/AA to +/-/1(Out1) -> >=<0 to 012/1(In1), Product1/2
  Product1/1 -> Transfer Fcn/1  "Mag_current"
  Cmd_Dir/1 -> 55/AA to +/-/1(In1)
  >=<0 to 012/1(Out1) -> Cmd_Dirr/1
  Transfer Fcn/1 -> "Cmd_Curr "/1

== system GS_model/Subsystem2/Subsystem/Actuator/Magnetorquer/Mt_MathModel/MtA3/Triggered Subsystem6 ==
  In1 : Inport
  Enable : EnablePort
  Out1 : Outport  InitialOutput=0
  wires:
  In1/1 -> Out1/1

== system GS_model/Subsystem2/Subsystem/Actuator/Magnetorquer/Mt_MathModel/MtA4/>=<0 to 012 ==
  note: 2--负向
  note: 0
  note: 1--正向
  In1 : Inport
  Add1 : Sum  Inputs=+++
  Cast To Double : DataTypeConversion  OutDataTypeStr=double
  Cast To Double1 : DataTypeConversion  OutDataTypeStr=double
  Cast To Double2 : DataTypeConversion  OutDataTypeStr=double
  Compare To Zero : simulink/Logic and Bit Operations/Compare To Zero  relop=<  OutDataTypeStr=boolean
  Compare To Zero1 : simulink/Logic and Bit Operations/Compare To Zero  relop===  OutDataTypeStr=boolean
  Compare To Zero2 : simulink/Logic and Bit Operations/Compare To Zero  relop=>  OutDataTypeStr=boolean
  Constant1 : Constant
  Constant2 : Constant  Value=0
  Constant20 : Constant  Value=2
  Product1 : Product  SaturateOnIntegerOverflow=on  OutDataTypeStr=Inherit: Same as first input
  Product2 : Product  SaturateOnIntegerOverflow=on  OutDataTypeStr=Inherit: Same as first input
  Product6 : Product  SaturateOnIntegerOverflow=on  OutDataTypeStr=Inherit: Same as first input
  Out1 : Outport
  wires:
  Product2/1 -> Add1/3
  Cast To Double2/1 -> Product2/2
  Constant1/1 -> Product2/1
  Constant20/1 -> Product6/1
  Cast To Double1/1 -> Product1/2
  Cast To Double/1 -> Product6/2
  Add1/1 -> Out1/1
  Compare To Zero2/1 -> Cast To Double2/1
  Compare To Zero/1 -> Cast To Double/1
  In1/1 -> Compare To Zero/1, Compare To Zero1/1, Compare To Zero2/1
  Constant2/1 -> Product1/1
  Compare To Zero1/1 -> Cast To Double1/1
  Product6/1 -> Add1/1
  Product1/1 -> Add1/2

== system GS_model/Subsystem2/Subsystem/Actuator/Magnetorquer/Mt_MathModel/MtA4/If Action Subsystem3 ==
  In1 : Inport
  Action Port : ActionPort  ActionType=else
  Out1 : Outport
  wires:
  In1/1 -> Out1/1

== system GS_model/Subsystem2/Subsystem/Actuator/Magnetorquer/Mt_MathModel/MtA4/If Action Subsystem4 ==
  In1 : Inport
  Action Port : ActionPort  ActionType=then
  Out1 : Outport
  wires:
  In1/1 -> Out1/1

== system GS_model/Subsystem2/Subsystem/Actuator/Magnetorquer/Mt_MathModel/MtA4/Mag_CmdCal ==
  Cmd_Dir : Inport
  Cmd_Cur : Inport  Port=2
  55/AA to +/- : Subsystem
  >=<0 to 012 : Subsystem
  Product1 : Product
  Transfer Fcn : TransferFcn  Denominator=[Tao_Mt/3 1]
  "Cmd_Curr " : Outport
  Cmd_Dirr : Outport  Port=2
  wires:
  Transfer Fcn/1 -> "Cmd_Curr "/1
  >=<0 to 012/1(Out1) -> Cmd_Dirr/1
  Cmd_Dir/1 -> 55/AA to +/-/1(In1)
  Product1/1 -> Transfer Fcn/1  "Mag_current"
  55/AA to +/-/1(Out1) -> Product1/2, >=<0 to 012/1(In1)
  Cmd_Cur/1 -> Product1/1

== system GS_model/Subsystem2/Subsystem/Actuator/Magnetorquer/Mt_MathModel/MtA4/Triggered Subsystem6 ==
  In1 : Inport
  Enable : EnablePort
  Out1 : Outport  InitialOutput=0
  wires:
  In1/1 -> Out1/1

== system GS_model/Subsystem2/Subsystem/Actuator/Magnetorquer/Mt_MathModel/MtA5/>=<0 to 012 ==
  note: 1--正向
  note: 0
  note: 2--负向
  In1 : Inport
  Add1 : Sum  Inputs=+++
  Cast To Double : DataTypeConversion  OutDataTypeStr=double
  Cast To Double1 : DataTypeConversion  OutDataTypeStr=double
  Cast To Double2 : DataTypeConversion  OutDataTypeStr=double
  Compare To Zero : simulink/Logic and Bit Operations/Compare To Zero  relop=<  OutDataTypeStr=boolean
  Compare To Zero1 : simulink/Logic and Bit Operations/Compare To Zero  relop===  OutDataTypeStr=boolean
  Compare To Zero2 : simulink/Logic and Bit Operations/Compare To Zero  relop=>  OutDataTypeStr=boolean
  Constant1 : Constant
  Constant2 : Constant  Value=0
  Constant20 : Constant  Value=2
  Product1 : Product  SaturateOnIntegerOverflow=on  OutDataTypeStr=Inherit: Same as first input
  Product2 : Product  SaturateOnIntegerOverflow=on  OutDataTypeStr=Inherit: Same as first input
  Product6 : Product  SaturateOnIntegerOverflow=on  OutDataTypeStr=Inherit: Same as first input
  Out1 : Outport
  wires:
  Product1/1 -> Add1/2
  Product6/1 -> Add1/1
  Compare To Zero1/1 -> Cast To Double1/1
  Constant2/1 -> Product1/1
  In1/1 -> Compare To Zero2/1, Compare To Zero1/1, Compare To Zero/1
  Compare To Zero/1 -> Cast To Double/1
  Compare To Zero2/1 -> Cast To Double2/1
  Add1/1 -> Out1/1
  Cast To Double/1 -> Product6/2
  Cast To Double1/1 -> Product1/2
  Constant20/1 -> Product6/1
  Constant1/1 -> Product2/1
  Cast To Double2/1 -> Product2/2
  Product2/1 -> Add1/3

== system GS_model/Subsystem2/Subsystem/Actuator/Magnetorquer/Mt_MathModel/MtA5/If Action Subsystem3 ==
  In1 : Inport
  Action Port : ActionPort  ActionType=else
  Out1 : Outport
  wires:
  In1/1 -> Out1/1

== system GS_model/Subsystem2/Subsystem/Actuator/Magnetorquer/Mt_MathModel/MtA5/If Action Subsystem4 ==
  In1 : Inport
  Action Port : ActionPort  ActionType=then
  Out1 : Outport
  wires:
  In1/1 -> Out1/1

== system GS_model/Subsystem2/Subsystem/Actuator/Magnetorquer/Mt_MathModel/MtA5/Mag_CmdCal ==
  Cmd_Dir : Inport
  Cmd_Cur : Inport  Port=2
  55/AA to +/- : Subsystem
  >=<0 to 012 : Subsystem
  Product1 : Product
  Transfer Fcn : TransferFcn  Denominator=[Tao_Mt/3 1]
  "Cmd_Curr " : Outport
  Cmd_Dirr : Outport  Port=2
  wires:
  Cmd_Cur/1 -> Product1/1
  55/AA to +/-/1(Out1) -> >=<0 to 012/1(In1), Product1/2
  Product1/1 -> Transfer Fcn/1  "Mag_current"
  Cmd_Dir/1 -> 55/AA to +/-/1(In1)
  >=<0 to 012/1(Out1) -> Cmd_Dirr/1
  Transfer Fcn/1 -> "Cmd_Curr "/1

== system GS_model/Subsystem2/Subsystem/Actuator/Magnetorquer/Mt_MathModel/MtA5/Triggered Subsystem6 ==
  In1 : Inport
  Enable : EnablePort
  Out1 : Outport  InitialOutput=0
  wires:
  In1/1 -> Out1/1

== system GS_model/Subsystem2/Subsystem/Actuator/Magnetorquer/Mt_MathModel/MtA6/>=<0 to 012 ==
  note: 2--负向
  note: 0
  note: 1--正向
  In1 : Inport
  Add1 : Sum  Inputs=+++
  Cast To Double : DataTypeConversion  OutDataTypeStr=double
  Cast To Double1 : DataTypeConversion  OutDataTypeStr=double
  Cast To Double2 : DataTypeConversion  OutDataTypeStr=double
  Compare To Zero : simulink/Logic and Bit Operations/Compare To Zero  relop=<  OutDataTypeStr=boolean
  Compare To Zero1 : simulink/Logic and Bit Operations/Compare To Zero  relop===  OutDataTypeStr=boolean
  Compare To Zero2 : simulink/Logic and Bit Operations/Compare To Zero  relop=>  OutDataTypeStr=boolean
  Constant1 : Constant
  Constant2 : Constant  Value=0
  Constant20 : Constant  Value=2
  Product1 : Product  SaturateOnIntegerOverflow=on  OutDataTypeStr=Inherit: Same as first input
  Product2 : Product  SaturateOnIntegerOverflow=on  OutDataTypeStr=Inherit: Same as first input
  Product6 : Product  SaturateOnIntegerOverflow=on  OutDataTypeStr=Inherit: Same as first input
  Out1 : Outport
  wires:
  Product2/1 -> Add1/3
  Cast To Double2/1 -> Product2/2
  Constant1/1 -> Product2/1
  Constant20/1 -> Product6/1
  Cast To Double1/1 -> Product1/2
  Cast To Double/1 -> Product6/2
  Add1/1 -> Out1/1
  Compare To Zero2/1 -> Cast To Double2/1
  Compare To Zero/1 -> Cast To Double/1
  In1/1 -> Compare To Zero/1, Compare To Zero1/1, Compare To Zero2/1
  Constant2/1 -> Product1/1
  Compare To Zero1/1 -> Cast To Double1/1
  Product6/1 -> Add1/1
  Product1/1 -> Add1/2

== system GS_model/Subsystem2/Subsystem/Actuator/Magnetorquer/Mt_MathModel/MtA6/If Action Subsystem3 ==
  In1 : Inport
  Action Port : ActionPort  ActionType=else
  Out1 : Outport
  wires:
  In1/1 -> Out1/1

== system GS_model/Subsystem2/Subsystem/Actuator/Magnetorquer/Mt_MathModel/MtA6/If Action Subsystem4 ==
  In1 : Inport
  Action Port : ActionPort  ActionType=then
  Out1 : Outport
  wires:
  In1/1 -> Out1/1

== system GS_model/Subsystem2/Subsystem/Actuator/Magnetorquer/Mt_MathModel/MtA6/Mag_CmdCal ==
  Cmd_Dir : Inport
  Cmd_Cur : Inport  Port=2
  55/AA to +/- : Subsystem
  >=<0 to 012 : Subsystem
  Product1 : Product
  Transfer Fcn : TransferFcn  Denominator=[Tao_Mt/3 1]
  "Cmd_Curr " : Outport
  Cmd_Dirr : Outport  Port=2
  wires:
  Transfer Fcn/1 -> "Cmd_Curr "/1
  >=<0 to 012/1(Out1) -> Cmd_Dirr/1
  Cmd_Dir/1 -> 55/AA to +/-/1(In1)
  Product1/1 -> Transfer Fcn/1  "Mag_current"
  55/AA to +/-/1(Out1) -> Product1/2, >=<0 to 012/1(In1)
  Cmd_Cur/1 -> Product1/1

== system GS_model/Subsystem2/Subsystem/Actuator/Magnetorquer/Mt_MathModel/MtA6/Triggered Subsystem6 ==
  In1 : Inport
  Enable : EnablePort
  Out1 : Outport  InitialOutput=0
  wires:
  In1/1 -> Out1/1

== system GS_model/Subsystem2/Subsystem/PhysicsModel/Environment/Air Torque Subsystem/satalite board/+Y SolarPanel ==
  vs(b) : Inport
  Fa' : Inport  Port=2
  "Abp " : Inport  Port=3
  Cent : Inport  Port=4
  3x3 Cross Product1 : sharedutil/3x3 Cross Product  aMode=aMode
      settings: SourceProductBaseCode=AE,PW,MT,VE,VP
  Compute press of sun radiation1 : Subsystem  TreatAsAtomicUnit=on
  compute centroi 1 : Subsystem  TreatAsAtomicUnit=on
  "T_panel " : Outport
  "F_panel " : Outport  Port=2
  wires:
  Compute press of sun radiation1/1("F_panel ") -> 3x3 Cross Product1/2, "F_panel "/1
  "Abp "/1 -> Compute press of sun radiation1/1("Abp "), compute centroi 1/2(Abp_PY)
  3x3 Cross Product1/1 -> "T_panel "/1
  vs(b)/1 -> Compute press of sun radiation1/2(vs(b))
  Fa'/1 -> Compute press of sun radiation1/3(Fa')
  Cent/1 -> compute centroi 1/1(Cent)
  compute centroi 1/1(r) -> 3x3 Cross Product1/1

== system GS_model/Subsystem2/Subsystem/PhysicsModel/Environment/Air Torque Subsystem/satalite board/-Y SolarPanel ==
  vs(b) : Inport
  Fa' : Inport  Port=2
  "Abp " : Inport  Port=3
  Cent : Inport  Port=4
  3x3 Cross Product1 : sharedutil/3x3 Cross Product  aMode=aMode
      settings: SourceProductBaseCode=AE,PW,MT,VE,VP
  Compute press of sun radiation : Subsystem  TreatAsAtomicUnit=on
  compute centroi 1 : Subsystem  TreatAsAtomicUnit=on
  "T_panel " : Outport
  "F_panel " : Outport  Port=2
  wires:
  Fa'/1 -> Compute press of sun radiation/3(Fa')
  vs(b)/1 -> Compute press of sun radiation/2(vs(b))
  3x3 Cross Product1/1 -> "T_panel "/1
  "Abp "/1 -> compute centroi 1/2(Abp_NY), Compute press of sun radiation/1("Abp ")
  Compute press of sun radiation/1("F_panel ") -> "F_panel "/1, 3x3 Cross Product1/2
  Cent/1 -> compute centroi 1/1(Cent)
  compute centroi 1/1(r) -> 3x3 Cross Product1/1

== system GS_model/Subsystem2/Subsystem/PhysicsModel/Environment/Air Torque Subsystem/satalite board/Torque from  board perpendicular to z axis  ==
  "[Vs]b_nor" : Inport
  Fa' : Inport  Port=2
  Cent : Inport  Port=3
  3x3 Cross Product : sharedutil/3x3 Cross Product  aMode=aMode
      settings: SourceProductBaseCode=AE,PW,MT,VE,VP
  Compute press of sun radiation : Subsystem  TreatAsAtomicUnit=on
  compute centroi 1 : Subsystem  TreatAsAtomicUnit=on
  Tz : Outport
  Fz : Outport  Port=2
  wires:
  compute centroi 1/1(r_z) -> 3x3 Cross Product/1
  3x3 Cross Product/1 -> Tz/1
  Compute press of sun radiation/1(Fz) -> 3x3 Cross Product/2, Fz/1
  "[Vs]b_nor"/1 -> compute centroi 1/1(Orientation), Compute press of sun radiation/1("[Vs]b_nor")
  Fa'/1 -> Compute press of sun radiation/2(Fa')
  Cent/1 -> compute centroi 1/2(Cent)

== system GS_model/Subsystem2/Subsystem/PhysicsModel/Environment/Air Torque Subsystem/satalite board/Torque from board perpendicular to x axis ==
  vs(b) : Inport
  Fa' : Inport  Port=2
  Cent : Inport  Port=3
  3x3 Cross Product : sharedutil/3x3 Cross Product  aMode=aMode
      settings: SourceProductBaseCode=AE,PW,MT,VE,VP
  Compute press of sun radiation : Subsystem  TreatAsAtomicUnit=on
  compute centroi 1 : Subsystem  TreatAsAtomicUnit=on
  Tx : Outport
  Fx : Outport  Port=2
  wires:
  compute centroi 1/1(r_x) -> 3x3 Cross Product/1
  vs(b)/1 -> compute centroi 1/1(Orientation), Compute press of sun radiation/1(Vs(b))
  3x3 Cross Product/1 -> Tx/1
  Compute press of sun radiation/1(Fx) -> 3x3 Cross Product/2, Fx/1
  Fa'/1 -> Compute press of sun radiation/2(Fa')
  Cent/1 -> compute centroi 1/2(Cent)

== system GS_model/Subsystem2/Subsystem/PhysicsModel/Environment/Air Torque Subsystem/satalite board/Torque from board perpendicular to y axis ==
  vs(b) : Inport
  Fa' : Inport  Port=2
  Cent : Inport  Port=3
  3x3 Cross Product : sharedutil/3x3 Cross Product  aMode=aMode
      settings: SourceProductBaseCode=AE,PW,MT,VE,VP
  Compute press of sun radiation : Subsystem  TreatAsAtomicUnit=on
  compute centroi 1 : Subsystem  TreatAsAtomicUnit=on
  Ty : Outport
  Fy : Outport  Port=2
  wires:
  compute centroi 1/1(r_y) -> 3x3 Cross Product/1
  3x3 Cross Product/1 -> Ty/1
  Compute press of sun radiation/1(Fy) -> 3x3 Cross Product/2, Fy/1
  vs(b)/1 -> compute centroi 1/1(Orientation), Compute press of sun radiation/1(vs(b))
  Fa'/1 -> Compute press of sun radiation/2(Fa')
  Cent/1 -> compute centroi 1/2(Cent)

== system GS_model/Subsystem2/Subsystem/PhysicsModel/Environment/MagneticCal/Subsystem1/Aop1 ==
  In1 : Inport
  Constant : Constant
  Constant1 : Constant  Value=0
  Gain1 : Gain  Gain=-1
  Mux2 : Mux  Inputs=9
  Reshape : Reshape  OutputDimensionality=Customize  OutputDimensions=[3,3]
  Trigonometric Function : Trigonometry
  Trigonometric Function1 : Trigonometry  Operator=cos
  Out1 : Outport
  wires:
  Trigonometric Function/1 -> Gain1/1, Mux2/2
  Trigonometric Function1/1 -> Mux2/5, Mux2/1
  In1/1 -> Trigonometric Function/1, Trigonometric Function1/1
  Constant1/1 -> Mux2/3, Mux2/6, Mux2/7, Mux2/8
  Constant/1 -> Mux2/9
  Mux2/1 -> Reshape/1
  Reshape/1 -> Out1/1
  Gain1/1 -> Mux2/4

== system GS_model/Subsystem2/Subsystem/PhysicsModel/Environment/MagneticCal/Subsystem1/If Action Subsystem ==
  In1 : Inport
  Action Port : ActionPort  ActionType=then
  Out1 : Outport
  wires:
  In1/1 -> Out1/1

== system GS_model/Subsystem2/Subsystem/PhysicsModel/Environment/MagneticCal/Subsystem1/If Action Subsystem1 ==
  In1 : Inport
  Action Port : ActionPort  ActionType=else
  Constant : Constant  Value=pi
  Sum : Sum  Inputs=|-+
  Out1 : Outport
  wires:
  Sum/1 -> Out1/1
  In1/1 -> Sum/1
  Constant/1 -> Sum/2

== system GS_model/Subsystem2/Subsystem/PhysicsModel/Environment/Sun  press torque/Panel Angle/If Action Subsystem ==
  In1 : Inport
  Action Port : ActionPort  ActionType=then
  Constant : Constant  Value=2*pi
  Sum : Sum  Inputs=|-+  SaturateOnIntegerOverflow=on
  Out1 : Outport
  wires:
  Sum/1 -> Out1/1
  In1/1 -> Sum/1
  Constant/1 -> Sum/2

== system GS_model/Subsystem2/Subsystem/PhysicsModel/Environment/Sun  press torque/Panel Angle/If Action Subsystem1 ==
  In1 : Inport
  Action Port : ActionPort  ActionType=else
  Out1 : Outport
  wires:
  In1/1 -> Out1/1

== system GS_model/Subsystem2/Subsystem/PhysicsModel/Environment/Sun  press torque/Sun  press torque2/If Action Subsystem3 ==
  Action Port : ActionPort  ActionType=else
  Constant2 : Constant  Value=zeros(3,1)
  Constant3 : Constant  Value=zeros(3,1)
  F_sun : Outport  InitialOutput=zeros(3,1)
  T_sun : Outport  Port=2  InitialOutput=zeros(3,1)
  wires:
  Constant2/1 -> T_sun/1
  Constant3/1 -> F_sun/1

== system GS_model/Subsystem2/Subsystem/PhysicsModel/Environment/Sun  press torque/Sun  press torque2/Sun  press torque ==
  sun(b) : Inport
  Abp_PY : Inport  Port=2
  Abp_NY : Inport  Port=3
  Cent : Inport  Port=4
  UnlockSpread : Inport  Port=5
  TC_SunPressCoeff : Inport  Port=6
  Action Port : ActionPort  ActionType=then
  +Y SunPanel : Subsystem  TreatAsAtomicUnit=on
  -Y SunPanel : Subsystem  TreatAsAtomicUnit=on
  Demux : Demux  Outputs=2
  Product{1..4} (4 alike) : Product  SaturateOnIntegerOverflow=on  OutDataTypeStr=Inherit: Same as first input
  Sum1 : Sum  Inputs=+++
  Sum2 : Sum  Inputs=+++
  Torque from   satalite board : Subsystem
  T_sun : Outport
  F_sun : Outport  Port=2
  wires:
  sun(b)/1 -> Torque from   satalite board/1(SunOrientation), -Y SunPanel/1(Sun(b)), +Y SunPanel/1(Sun(b))
  Torque from   satalite board/2(F_board) -> Sum2/1
  Sum2/1 -> F_sun/1
  Torque from   satalite board/1(T_board) -> Sum1/1
  Sum1/1 -> T_sun/1
  Cent/1 -> -Y SunPanel/2(Cent), +Y SunPanel/2(Cent), Torque from   satalite board/2(Cent)
  +Y SunPanel/2(F) -> Product3/1
  +Y SunPanel/1(T) -> Product1/1
  Abp_PY/1 -> +Y SunPanel/3(Abp)
  -Y SunPanel/2(F) -> Product4/2
  -Y SunPanel/1(T) -> Product2/2
  Abp_NY/1 -> -Y SunPanel/3(Abp)
  Product4/1 -> Sum2/3
  Product2/1 -> Sum1/3
  UnlockSpread/1 -> Demux/1
  Demux/1 -> Product1/2, Product3/2
  Demux/2 -> Product2/1, Product4/1
  TC_SunPressCoeff/1 -> -Y SunPanel/4(TC_SunPressCoeff), +Y SunPanel/4(TC_SunPressCoeff), Torque from   satalite board/3(TC_SunPressCoeff)
  Product3/1 -> Sum2/2
  Product1/1 -> Sum1/2

== system GS_model/Subsystem2/Subsystem/PhysicsModel/Orbit/Compute osculating elements/ /If Action Subsystem ==
  note: In+2pi, due to OMG's Range=[0 2*pi],
      | and atan2's Range=[-pi pi]
  In1 : Inport
  Action Port : ActionPort  ActionType=then
  Constant : Constant  Value=2*pi
  Sum : Sum  Inputs=|++  SaturateOnIntegerOverflow=on
  Out1 : Outport
  wires:
  In1/1 -> Sum/1
  Sum/1 -> Out1/1
  Constant/1 -> Sum/2

== system GS_model/Subsystem2/Subsystem/PhysicsModel/Orbit/Compute osculating elements/ /If Action Subsystem1 ==
  In1 : Inport
  Action Port : ActionPort  ActionType=else
  Out1 : Outport
  wires:
  In1/1 -> Out1/1

== system GS_model/Subsystem2/Subsystem/PhysicsModel/Orbit/Compute osculating elements/     /If Action Subsystem2 ==
  In1 : Inport
  Action Port : ActionPort  ActionType=then
  Out1 : Outport
  wires:
  In1/1 -> Out1/1

== system GS_model/Subsystem2/Subsystem/PhysicsModel/Orbit/Compute osculating elements/     /If Action Subsystem3 ==
  In1 : Inport
  Action Port : ActionPort  ActionType=else
  Constant : Constant  Value=2*pi
  Sum : Sum  Inputs=|+-  SaturateOnIntegerOverflow=on
  Out1 : Outport
  wires:
  Sum/1 -> Out1/1
  In1/1 -> Sum/2
  Constant/1 -> Sum/1

== system GS_model/Subsystem2/Subsystem/PhysicsModel/Orbit/Compute osculating elements/   1/If Action Subsystem ==
  In1 : Inport
  Action Port : ActionPort  ActionType=then
  Out1 : Outport
  wires:
  In1/1 -> Out1/1

== system GS_model/Subsystem2/Subsystem/PhysicsModel/Orbit/Compute osculating elements/   1/If Action Subsystem1 ==
  In1 : Inport
  Action Port : ActionPort  ActionType=else
  Constant : Constant  Value=2*pi
  Sum : Sum  Inputs=|++  SaturateOnIntegerOverflow=on
  Out1 : Outport
  wires:
  Sum/1 -> Out1/1
  In1/1 -> Sum/2
  Constant/1 -> Sum/1
